simulink model "purePursuitCurveHighVel"  (R2020a)
settings: Solver=VariableStepAuto  StartTime=0.0  StopTime=Ts  RelTol=1e-3
PreLoadFcn:
  | setUpPurePursuitCurveHighVel
model workspace (MAT data in the model file):
  firstWarning = 0
  originalScenarioChecksum = 'F73A6DA3C723D3CA73A6F931B7A52A9C'
values from neighbouring files (symbols this model uses):
  L = 3    [setUpPurePursuitCurveHighVel.m]
  ld = 7    [setUpPurePursuitCurveHighVel.m]
  psi_o = 0    [setUpPurePursuitCurveHighVel.m]
  s = size(xRef)    [setUpPurePursuitCurveHighVel.m]
  vel = lookUpt(2:30,2:20)    [setUpPurePursuitCurveHighVel.m]
  X_o = refPose(1,1)    [setUpPurePursuitCurveHighVel.m]
  xlt = lookUpt(2:30,1)    [setUpPurePursuitCurveHighVel.m]
  xRef = refPose(:,1)    [setUpPurePursuitCurveHighVel.m]
  Y_o = -refPose(1,2)    [setUpPurePursuitCurveHighVel.m]
  ylt = lookUpt(1,2:20)    [setUpPurePursuitCurveHighVel.m]
  yRef = -refPose(:,2)    [setUpPurePursuitCurveHighVel.m]
libraries: autolibutils x4, autolibshared x3, vehdynlibviscommon x1, robotalgslib x1, simulink x1
(part 3 of 3)

== system purePursuitCurveHighVel/Powertrain & Driveline/Driveline/FWD ==
  TPowertrain : Inport
  FWD : Gain  Gain=[1;1;0;0]
  TAxles : Outport  VectorParamsAs1DForOutWhenUnconnected=off
  wires:
  FWD/1 -> TAxles/1
  TPowertrain/1 -> FWD/1

== system purePursuitCurveHighVel/Powertrain & Driveline/Driveline/RWD ==
  TPowertrain : Inport
  RWD : Gain  Gain=[0;0;1;1]
  TAxles : Outport  VectorParamsAs1DForOutWhenUnconnected=off
  wires:
  TPowertrain/1 -> RWD/1
  RWD/1 -> TAxles/1
